simulink library "MSZSZ_MK"  (R2025a)
settings: Solver=VariableStepAuto  StartTime=0.0  StopTime=10.0  RelTol=1e-3
libraries: $bdroot x1
settings Model: Creator=Szalay  LastModifiedBy=Szalay

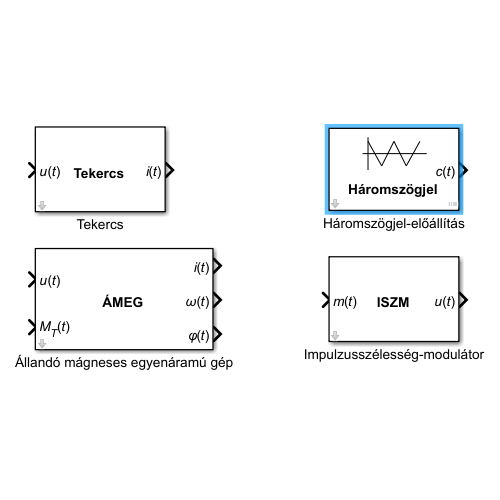
[thumbnail: Simulink's stored preview of the top-level diagram]
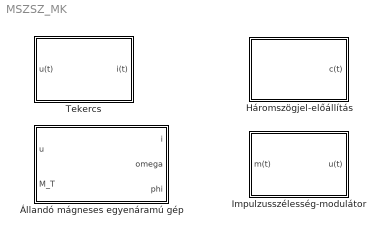
== system MSZSZ_MK ==
  Háromszögjel-előállítás : Subsystem  mask(Háromszögjel){A=1, f=10, B=0}
      mask prompts: A "Amplitúdó"; f "Frekvencia"; B "Középérték"
      mask help: Paraméterezhető háromszögjel-előállítás.
      mask DialogControl ParameterGroupVar Prompt: Beállítások
      mask Display:
      | % Felirat
      | text(0.5, 0.30, '\bfHáromszögjel', ...
      |     'HorizontalAlignment', 'center', ...
      |     'texmode', 'on' ...
      |     );
      | 
      | plot([25, 75]/100, (70 + [0, 0])/100);
      | plot([30, 30]/100, (70 + [-20, 20])/100);
      | plot([30, 40, 50, 60, 70]/100, (70 + [15, -15, 15, -15, 15])/100);
      | 
      | % Csatlakozók
      | port_label('output', 1, '{\itc}({\itt})', 'texmode', 'on');
  Impulzusszélesség-modulátor : Subsystem  mask(Impulzusszélesség-modulátor){U_T=12, f_ISZM=1000, T_D=1e-6}
      mask prompts: U_T "Tápfeszültség"; f_ISZM "Modulációs frekvencia"; T_D "Kapcsolási holtidő"
      mask help: Háromszög hordozójeles folytonos idejű ISZM.
      mask DialogControl ParameterGroupVar Prompt: Beállítások
      mask Display:
      | % Felirat
      | text(0.5, 0.5, '\bfISZM', ...
      |     'HorizontalAlignment', 'center', ...
      |     'texmode', 'on' ...
      |     );
      | 
      | % Csatlakozók
      | port_label('input', 1, '{\itm}({\itt})', 'texmode', 'on');
      | port_label('output', 1, '{\itu}({\itt})', 'texmode', 'on');
  Tekercs : Subsystem  mask(Tekercs){R=1, L=1e-3, i_0=-1}
      mask prompts: R "Ellenállás"; L "Induktivitás"; i_0 "Kezdeti áramerősség"
      mask help: Lineáris mágnesezésű tekercsmodell.
      mask DialogControl ParameterGroupVar Prompt: Modellparaméterek
      mask DialogControl Container3 Prompt: Kezdeti érték
      mask Display:
      | % Felirat
      | text(0.5, 0.5, '\bfTekercs', ...
      |     'HorizontalAlignment', 'center', ...
      |     'texmode', 'on' ...
      |     );
      | 
      | % Csatlakozók
      | port_label('input', 1, '{\itu}({\itt})', 'texmode', 'on');
      | port_label('output', 1, '{\iti}({\itt})', 'texmode', 'on');
  Állandó mágneses egyenáramú gép : Subsystem  mask(Állandó mágneses egyenáramú gép){R=212e-3, L=77e-6, k_T=23.4e-3, k_E=23.4e-3, J=102e-7, B=5.4932e-6, i_0=0, omega_0=0, phi_0=0}
      mask prompts: R "Ellenállás"; L "Induktivitás"; k_T "Nyomatékállandó"; k_E "Feszültségállandó"; J "Tehetetlenségi nyomaték"; B "Forgási súrlódási együttható"; i_0 "Kezdeti áramerősség"; omega_0 "Kezdeti szögsebesség"; phi_0 "Kezdeti szöghelyzet"
      mask help: Az állandó mágneses egyenáramú gép modellje alapértelmezetten a <i>Maxon&nbsp;DCX&nbsp;35&nbsp;L</i> 18&nbsp;V-os változata alapján paraméterezve.
      mask DialogControl Container4 Prompt: Modellparaméterek
      mask DialogControl ParameterGroupVar Prompt: Villamos áramköri részrendszer
      mask DialogControl Container6 Prompt: Mágnesköri gépállandók
      mask DialogControl Container7 Prompt: Forgó részrendszer
      mask DialogControl Container5 Prompt: Kezdeti értékek
      mask DialogControl Container8 Prompt: Villamos áramköri részrendszer
      mask DialogControl Container9 Prompt: Forgó részrendszer
      mask Display:
      | % Felirat
      | text(0.5, 0.5, '\bfÁMEG', ...
      |     'HorizontalAlignment', 'center', ...
      |     'texmode', 'on' ...
      |     );
      | 
      | % Csatlakozók
      | port_label('input', 1, '{\itu}({\itt})', 'texmode', 'on');
      | port_label('input', 2, '{\itM_T}({\itt})', 'texmode', 'on');
      | 
      | port_label('output', 1, '{\iti}({\itt})', 'texmode', 'on');
      | port_label('output', 2, '{\it\omega}({\itt})', 'texmode', 'on');
      | port_label('output', 3, '{\it\phi}({\itt})', 'texmode', 'on');

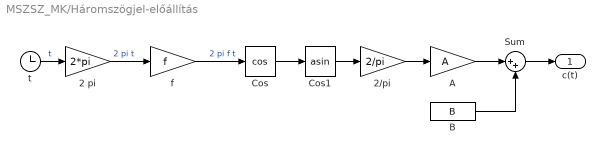
== system MSZSZ_MK/Háromszögjel-előállítás ==
  2 pi : Gain  Gain=2*pi
  2/pi : Gain  Gain=2/pi
  A : Gain  Gain=A
  B : Constant  Value=B
  Cos : Trigonometry  Operator=cos
  Cos1 : Trigonometry  Operator=asin
  Sum : Sum  Inputs=|++
  f : Gain  Gain=f
  t : Clock
  c(t) : Outport
  wires:
  Cos1/1 -> 2/pi/1
  Cos/1 -> Cos1/1
  2 pi/1 -> f/1  "2 pi t"
  f/1 -> Cos/1  "2 pi f t"
  t/1 -> 2 pi/1  "t"
  2/pi/1 -> A/1
  A/1 -> Sum/1
  Sum/1 -> c(t)/1
  B/1 -> Sum/2

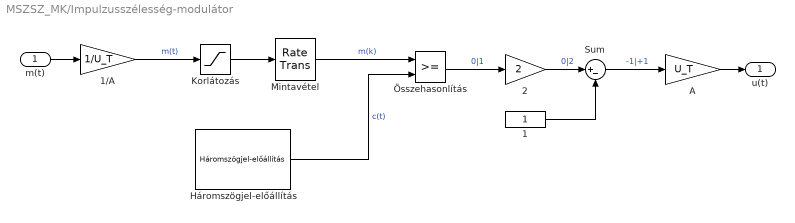
== system MSZSZ_MK/Impulzusszélesség-modulátor ==
  m(t) : Inport
  1 : Constant
  1/A : Gain  Gain=1/U_T
  2 : Gain  Gain=2
  A : Gain  Gain=U_T
  Háromszögjel-előállítás : $bdroot/Háromszögjel-előállítás  A=1  f=f_ISZM  B=0
  Korlátozás : Saturate  UpperLimit=1 - 2*T_D*f_ISZM  LowerLimit=-(1 - 2*T_D*f_ISZM)
  Mintavétel : RateTransition  OutPortSampleTime=1/f_ISZM/2
  Sum : Sum  Inputs=|+-
  Összehasonlítás : RelationalOperator  OutDataTypeStr=boolean  RndMeth=Simplest  InputSameDT=off
  u(t) : Outport
  wires:
  m(t)/1 -> 1/A/1
  Háromszögjel-előállítás/1 -> Összehasonlítás/2  "c(t)"
  Sum/1 -> A/1  "-1|+1"
  Mintavétel/1 -> Összehasonlítás/1  "m(k)"
  Összehasonlítás/1 -> 2/1  "0|1"
  2/1 -> Sum/1  "0|2"
  Korlátozás/1 -> Mintavétel/1
  1/1 -> Sum/2
  1/A/1 -> Korlátozás/1  "m(t)"
  A/1 -> u(t)/1

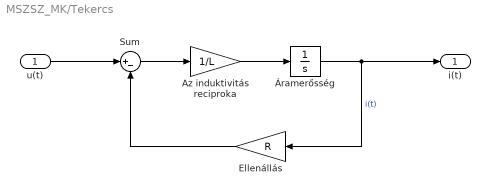
== system MSZSZ_MK/Tekercs ==
  u(t) : Inport
  Az induktivitás reciproka : Gain  Gain=1/L
  Ellenállás : Gain  Gain=R
  Sum : Sum  Inputs=|+-
  Áramerősség : Integrator  InitialCondition=i_0
  i(t) : Outport
  wires:
  Az induktivitás reciproka/1 -> Áramerősség/1
  Áramerősség/1 -> i(t)/1, Ellenállás/1  "i(t)"
  Sum/1 -> Az induktivitás reciproka/1
  Ellenállás/1 -> Sum/2
  u(t)/1 -> Sum/1

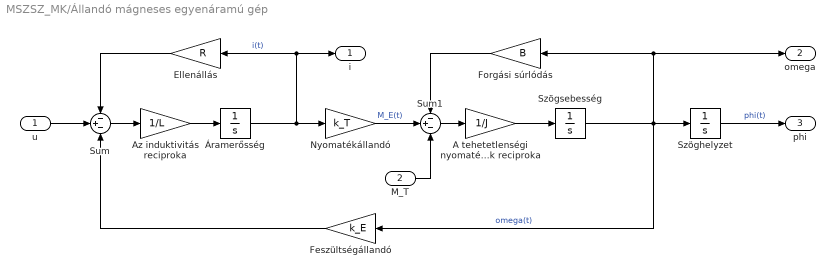
== system MSZSZ_MK/Állandó mágneses egyenáramú gép ==
  u : Inport
  M_T : Inport  Port=2
  A tehetetlenségi nyomaték reciproka : Gain  Gain=1/J
  Az induktivitás reciproka : Gain  Gain=1/L
  Ellenállás : Gain  Gain=R
  Feszültségállandó : Gain  Gain=k_E
  Forgási súrlódás : Gain  Gain=B
  Nyomatékállandó : Gain  Gain=k_T
  Sum : Sum  Inputs=-+-
  Sum1 : Sum  Inputs=-+-
  Szöghelyzet : Integrator  InitialCondition=phi_0
  Szögsebesség : Integrator  InitialCondition=omega_0
  Áramerősség : Integrator  InitialCondition=i_0
  i : Outport
  omega : Outport  Port=2
  phi : Outport  Port=3
  wires:
  Ellenállás/1 -> Sum/1
  Feszültségállandó/1 -> Sum/3
  A tehetetlenségi nyomaték reciproka/1 -> Szögsebesség/1
  Áramerősség/1 -> i/1, Ellenállás/1, Nyomatékállandó/1  "i(t)"
  Az induktivitás reciproka/1 -> Áramerősség/1
  Szögsebesség/1 -> Szöghelyzet/1, Feszültségállandó/1, Forgási súrlódás/1, omega/1  "omega(t)"
  Nyomatékállandó/1 -> Sum1/2  "M_E(t)"
  Sum1/1 -> A tehetetlenségi nyomaték reciproka/1
  Forgási súrlódás/1 -> Sum1/1
  Sum/1 -> Az induktivitás reciproka/1
  u/1 -> Sum/2
  M_T/1 -> Sum1/3
  Szöghelyzet/1 -> phi/1  "phi(t)"
